simulink model "IsolatedBatteryModel"  (R2022a)
settings: Solver=ode4  StartTime=0.0  StopTime=inf  FixedStep=1/180  RelTol=1e-3
undefined symbols (not defined in the file or in its folder): Batt
libraries: aerolibanimutils x1
settings Model: Creator=drimo  LastModifiedBy=drimo

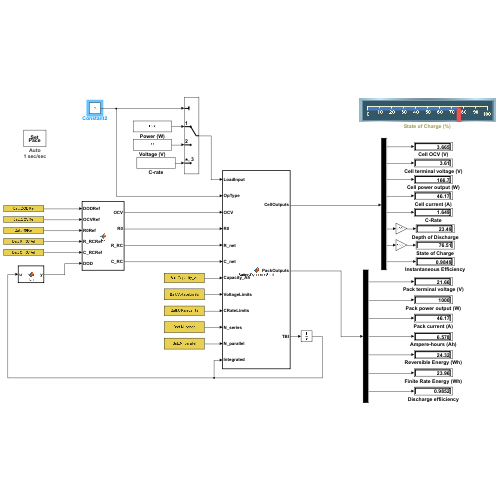
[thumbnail: Simulink's stored preview of the top-level diagram]
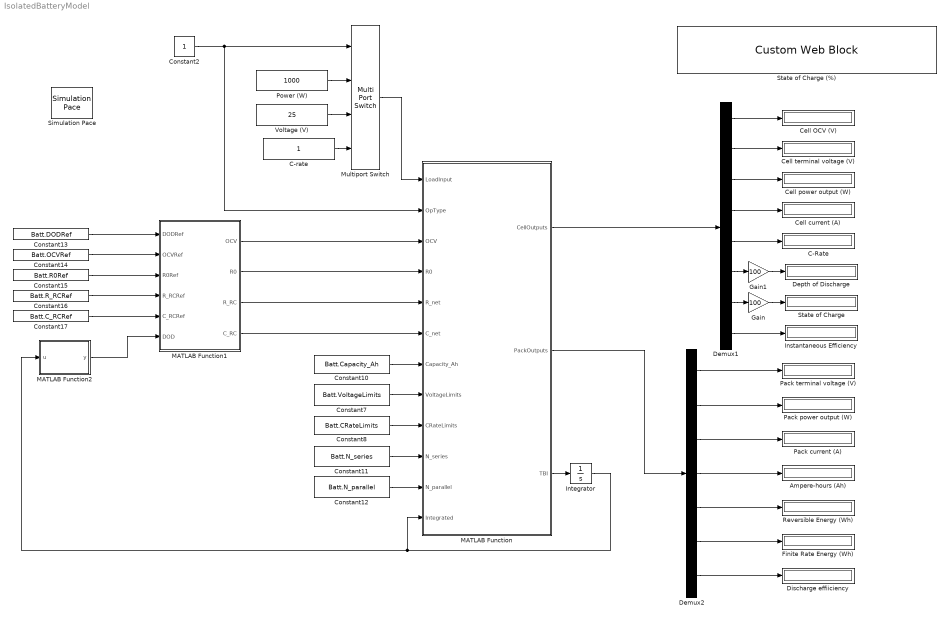
== system IsolatedBatteryModel ==
  Ampere-hours (Ah) : Display
  C-Rate : Display
  C-rate : Constant
  Cell OCV (V) : Display
  Cell current (A) : Display
  Cell power output (W) : Display
  Cell terminal voltage (V) : Display
  Constant10 : Constant  Value=Batt.Capacity_Ah
  Constant11 : Constant  Value=Batt.N_series
  Constant12 : Constant  Value=Batt.N_parallel
  Constant13 : Constant  Value=Batt.DODRef
  Constant14 : Constant  Value=Batt.OCVRef
  Constant15 : Constant  Value=Batt.R0Ref
  Constant16 : Constant  Value=Batt.R_RCRef
  Constant17 : Constant  Value=Batt.C_RCRef
  Constant2 : Constant
  Constant7 : Constant  Value=Batt.VoltageLimits
  Constant8 : Constant  Value=Batt.CRateLimits
  Demux1 : Demux  Outputs=8
  Demux2 : Demux  Outputs=7
  Depth of Discharge : Display
  Discharge effiiciency : Display
  Finite Rate Energy (Wh) : Display
  Gain : Gain  Gain=100
  Gain1 : Gain  Gain=100
  Instantaneous Efficiency : Display
  Integrator : Integrator  InitialCondition=[0,0,0,0,0]
  MATLAB Function : MATLAB Function  TreatAsAtomicUnit=on
  MATLAB Function1 : MATLAB Function  TreatAsAtomicUnit=on
  MATLAB Function2 : MATLAB Function  TreatAsAtomicUnit=on
  Multiport Switch : MultiPortSwitch  SaturateOnIntegerOverflow=off  InputSameDT=off
  Pack current (A) : Display
  Pack power output (W) : Display
  Pack terminal voltage (V) : Display
  Power (W) : Constant  Value=1000
  Reversible Energy (Wh) : Display
  Simulation Pace : aerolibanimutils/Simulation Pace  SimulationPace=1  SleepMode=Auto  OutputPaceError=off  SampleTime=1/30
  State of Charge : Display
  State of Charge (%) : CustomWebBlock  LabelPosition=Hide  ShowInitialText=on  Configuration="{\"type\":\"LinearGauge\",\"settings\":{\"BindingType\":\"signal\",\"backgroundColor\":[0,0,0,\"1\"],\"backgroundOffset\":0,\"backgroundOpacity\":1,\"fixedAspectRatio\":\"off\",\"orientation\":\"horizontal\",\"showBackgroundColor\":false,\"value\":0},\"components\":[{\"name\":\"LinearScaleComponent\",\"settings\":{\"bounds\":{\"max\":100,\"min\":0,\"tickInterval\":\"auto\"},\"internalTickHeightScaleFactor\":0.5,\"labelColor\":[255,255,200],\"labelFont\":{\"font\":\"Arial\",\"fontSize\":12},\"labelTransparency\":1,\"needleImage\":{\"size\":[21,75],\"src\":\"data:image/svg+xml;base64,PHN2ZyB4bWxucz0iaHR0cDovL3d3dy53My5vcmcvMjAwMC9zdmciIHhtbG5zOnhsaW5rPSJodHRwOi8vd3d3LnczLm9yZy8xOTk5L3hsaW5rIiB2aWV3Qm94PSIwIDAgMjEgNzUiPjxkZWZzPjxzdHlsZT4uY2xzLTF7ZmlsbDpub25lO30uY2xzLTJ7aXNvbGF0aW9uOmlzb2xhdGU7fS5jbHMtM3tjbGlwLXBhdGg6dXJsKCNjbGlwLXBhdGgpO30uY2xzLTR7b3BhY2l0eTowLjM7bWl4LWJsZW5kLW1vZGU6bXVsdGlwbHk7fS5jbHMtNXtmaWxsOiNlYjI2Mjk7fTwvc3R5bGU+PGNsaXBQYXRoIGlkPSJjbGlwLXBhdGgiIHRyYW5zZm9y ...(+1928 chars)\",\"srcOrientation\":\"horizontal\"},\"needleOffset\":[0,-0.007413509060955519],\"needleSize\":{\"height\":0.7589285714285714,\"width\":0.11955094537815127},\"position\":[0.06969246031746032,0.01995798319327731,0.9641544117647058,0.7998511904761905],\"referencePoint\":\"auto\",\"scaleColors\":[],\"scaleColorsSize\":0.2,\"scaleDirection\":\"LR\",\"showLabels\":1,\"showMinorTicks\":0,\"showSpanLine\":1,\"showTicks\":1,\"tickColor\":[252,252,197],\"tickTransparency\":1,\"valueBarColor\":[23,89,176],\"valueBarOffset\":0,\"valueBarSize\":0.23,\"valueBarTransparency\":1}},{\"name\":\"BackgroundImageComponent\",\"settings\":{\"image\":{\"size\":[380,101],\"src\":\"data:image/svg+xml;base64,PHN2ZyBpZD0iZnJhbWUiIHhtbG5zPSJodHRwOi8vd3d3LnczLm9yZy8yMDAwL3N2ZyIgeG1sbnM6eGxpbms9Imh0dHA6Ly93d3cudzMub3JnLzE5OTkveGxpbmsiIHZpZXdCb3g9IjAgMCAzODAgMTAxIj48ZGVmcz48c3R5bGU+LmNscy0xe2ZpbGw6IzAwMmI0Mjt9LmNscy0ye2ZpbGw6IzQyNzA4Mjt9LmNscy0ze2ZpbGw6dXJsKCNyYWRpYWwtZ3JhZGllbnQpO308L3N0eWxlPjxyYWRpYWxHcmFkaWVudCBpZD0icmFkaWFsLWdyYWRpZW50IiBjeD0iMTkwIiBjeT0iNTAuNSIgcj0iMjY5LjIxIiBncmFkaWVudFVuaXRzPSJ1c2VyU3BhY2VPblVzZSI+PHN0b3Agb2Zmc2V0PSIwLjAxIiBzdG9wLWNvbG9yPSIjM2U0ZjU4Ii8+PHN0b3Agb2Zmc2V0PSIwLjA2IiBzdG9wLWNvbG9yPSIjNDQ1NzYxIi8+PHN0b3Agb2Zmc2V0PSIwLjE1IiBzdG9wLWNvbG9yPSIjNTU2YTc2Ii8+PHN0b3Agb2Zmc2V0PSIwLjI1IiBzdG9wLWNvbG9yPSIjNmQ4ODk1Ii8+PHN0b3Agb2Zmc2V0PSIwLjM4IiBzdG9wLWNvbG9yPSIjOGZiMmMzIi8+PHN0b3Agb2Zmc2V0PSIwLjUyIiBzdG9wLWNvbG9yPSIjYjZlNGZhIi8+PHN0b3Agb2Zmc2V0PSIxIiBzdG9wLWNvbG9yPSIjMTU0NjU3Ii8+PC9yYWRpYWxHcmFkaWVudD48L2RlZnM+PGcgaWQ9IkxheWVyXzIiIGRhdGEtbmFtZT0iTGF5ZXIgMiI+PGcgaWQ9IkxheWVyXzEtMiIgZGF0YS1uYW1lPSJMYXllciAxLTIiPjxyZWN0IGlkPSJyZWN0MTAzNiIgY2xhc3M9ImNscy0xIiB4PSIxMSIgeT0iMTEiIHdpZHRoPSIzNTgiIGhlaWdodD0iNzkiLz48cGF0aCBpZD0icGF0aDEwMzgiIGNsYXNzPSJjbHMtMiIgZD0iTTgsOFY5M0gzNzJWOFpNMzY5LDkwSDExVjExSDM2OVoiLz48cGF0aCBpZD0icGF0aDEwNDAiIGNsYXNzPSJjbHMtMyIgZD0iTTAsMFYxMDFIMzgwVjBaTTM3Miw5M0g4VjhIMzcyWiIvPjwvZz48L2c+PC9zdmc+\",\"srcOrientation\":\"horizontal\"},\"position\":[0,0,1,1],\"scaleMode\":\"0\"}},{\"name\":\"ForegroundImageComponent\",\"settings\":{\"image\":{\"size\":[0,0],\"src\":\"default\",\"srcOrientation\":[]},\"isForeground\":1,\"position\":[0,0,1,1],\"scaleMode\":\"0\"}}]}"
  Voltage (V) : Constant  Value=25
  wires:
  Constant2/1 -> MATLAB Function/2(OpType), Multiport Switch/1
  Power (W)/1 -> Multiport Switch/2
  Constant7/1 -> MATLAB Function/8(VoltageLimits)
  Constant8/1 -> MATLAB Function/9(CRateLimits)
  Constant10/1 -> MATLAB Function/7(Capacity_Ah)
  MATLAB Function/3(TBI) -> Integrator/1
  Integrator/1 -> MATLAB Function2/1(u), MATLAB Function/12(Integrated)
  MATLAB Function/1(CellOutputs) -> Demux1/1
  MATLAB Function/2(PackOutputs) -> Demux2/1
  Constant11/1 -> MATLAB Function/10(N_series)
  Constant12/1 -> MATLAB Function/11(N_parallel)
  Constant13/1 -> MATLAB Function1/1(DODRef)
  Constant14/1 -> MATLAB Function1/2(OCVRef)
  Constant15/1 -> MATLAB Function1/3(R0Ref)
  Constant16/1 -> MATLAB Function1/4(R_RCRef)
  Constant17/1 -> MATLAB Function1/5(C_RCRef)
  MATLAB Function1/1(OCV) -> MATLAB Function/3(OCV)
  MATLAB Function1/2(R0) -> MATLAB Function/4(R0)
  MATLAB Function1/3(R_RC) -> MATLAB Function/5(R_net)
  MATLAB Function1/4(C_RC) -> MATLAB Function/6(C_net)
  Multiport Switch/1 -> MATLAB Function/1(LoadInput)
  Voltage (V)/1 -> Multiport Switch/3
  C-rate/1 -> Multiport Switch/4
  Demux1/1 -> Cell OCV (V)/1
  Demux1/2 -> Cell terminal voltage (V)/1
  Demux1/3 -> Cell power output (W)/1
  Demux1/4 -> Cell current (A)/1
  Demux1/5 -> C-Rate/1
  Demux1/6 -> Gain1/1
  Demux1/7 -> Gain/1
  Demux1/8 -> Instantaneous Efficiency/1
  Demux2/1 -> Pack terminal voltage (V)/1
  Demux2/2 -> Pack power output (W)/1
  Demux2/3 -> Pack current (A)/1
  Gain/1 -> State of Charge/1
  Demux2/4 -> Ampere-hours (Ah)/1
  Demux2/5 -> Reversible Energy (Wh)/1
  MATLAB Function2/1(y) -> MATLAB Function1/6(DOD)
  Demux2/6 -> Finite Rate Energy (Wh)/1
  Demux2/7 -> Discharge effiiciency/1
  Gain1/1 -> Depth of Discharge/1

== matlab function IsolatedBatteryModel/MATLAB Function1 ==
  data: DODRef input; OCVRef input; OCV output; R0Ref input; R_RCRef input; C_RCRef input; DOD input; R0 output; R_RC output; C_RC output
function [OCV, R0, R_RC, C_RC] = fcn(DODRef, OCVRef, R0Ref, R_RCRef, C_RCRef, DOD)


DODRef = DODRef';
OCVRef = OCVRef';
R0Ref = R0Ref';
R_RCRef = R_RCRef';
C_RCRef = C_RCRef';

IndexNum = 1:1:length(DODRef);

% Find the indices bracketing the incoming DOD value
inds = find(DOD<DODRef);
inds(isempty(inds)) = max(IndexNum);
ind_high = inds(1);
ind_low = max(1,ind_high-1);
II = ind_low + min(1, (DOD - DODRef(ind_low))/(DODRef(ind_high)-DODRef(ind_low)));
IQ = II-ind_low;


OCV = OCVRef(:,ind_low) + IQ * (OCVRef(:,ind_high) - OCVRef(:,ind_low));
R0 = R0Ref(:,ind_low) + IQ * (R0Ref(:,ind_high) - R0Ref(:,ind_low));
R_RC = R_RCRef(:,ind_low) + IQ * (R_RCRef(:,ind_high) - R_RCRef(:,ind_low));
C_RC = C_RCRef(:,ind_low) + IQ * (C_RCRef(:,ind_high) - C_RCRef(:,ind_low));

== matlab function IsolatedBatteryModel/MATLAB Function ==
  data: LoadInput input; CellOutputs output; PackOutputs output; OpType input; OCV input; R0 input; R_net input; C_net input; Capacity_Ah input; VoltageLimits input; CRateLimits input; N_series input; N_parallel input; TBI output; Integrated input
function [CellOutputs, PackOutputs, TBI] = BatteryDynamicsShell(LoadInput, OpType, OCV, R0, R_net, C_net, Capacity_Ah, VoltageLimits, CRateLimits, N_series, N_parallel, Integrated)

% coder.extrinsic('BatteryDynamics.m')

BattParams.Capacity_Ah = Capacity_Ah;
BattParams.VoltageLimits = VoltageLimits;
BattParams.CRateLimits = CRateLimits;
BattParams.N_series = N_series;
BattParams.N_parallel = N_parallel;

[CellOutputs, PackOutputs, TBI] = BatteryDynamics(LoadInput, OpType, OCV, R0, R_net, C_net, BattParams, Integrated);

== matlab function IsolatedBatteryModel/MATLAB Function2 ==
  data: u input; y output
function y = fcn(u)

y = u(1);
